simulink model "F16ASYM_Controlled_AoA"  (R2012b)
settings: Solver=ode3  SolverMode=SingleTasking  StartTime=0.0  StopTime=inf  FixedStep=T_sim  RelTol=1e-3
InitFcn:
  | load('NN_c_weights_Last_stable.mat')
values from neighbouring files (symbols this model uses):
  K_b_AoA = params(3)    [Cost_function.m]
  K_b_q = params(4)    [Cost_function.m]
  learning = 20    [Scheduling_desing.m]
  Model_used_flag = 1    [Scheduling_desing.m]
  reg_param = 0.5    [Scheduling_desing.m]
  T_sim = 0.02    [Scheduling_desing.m]
  tau_AoA = params(1)    [Cost_function.m]
  tau_q = params(2)    [Cost_function.m]
  Theta_1_roll_last = [0.00183613313267 0.00115998993235 0.0006676025148 0.00194921904952 0.00134963559861 0.00034352059664 0.000447169388141 0.00146749660935 0.00110199952389 7.77922383894e-05 0.00109492833348 0.00192687590535 ... (360 elements, 30x12)]    [NN_i_weights_LAST_STABLE.mat]
  Theta_2_roll_last = [0.000469743069697 0.000355923851088 0.00180035760697 0.00191855117771 0.00118851504447 0.0013331642065 0.0013164316578 0.000643981263341 0.00176817665434 0.000113802099363 0.000426534542462 0.00113815782354 ... (620 elements, 20x31)]    [NN_i_weights_LAST_STABLE.mat]
  Theta_3_roll_last = [9.62071520568e-05 -0.000389870886846 2.08260845013e-05 0.000140787743673 -0.000917525755397 -0.0014324207578 -0.00154701573815 -0.00131544476264 -0.00101205584381 5.06515794689e-05 -0.00111443483676 -0.00143957416141 ... (21 elements, 1x21)]    [NN_i_weights_LAST_STABLE.mat]
  V_long_lastA_w_z = [0.352826086601 -0.253633004548 -0.642535042878 0.237749930435 -0.618390629538 0.858074761295 0.268211230628 -0.448715080196 -0.0406384631192 0.401147605577 0.60598427709 0.0500551915851 ... (300 elements, 30x10)]    [NN_i_weights_LAST_STABLE.mat]
  V_long_lastAoA = [0.0774300162379 0.0911421319631 0.0352371192557 0.0542170286952 0.0651171200844 0.0177112012707 0.0982957728448 0.000259994642558 0.0194724569123 0.0466321328252 0.0556687953852 0.0252668067142 ... (300 elements, 30x10)]    [NN_i_weights_LAST_STABLE.mat]
  V_roll_last = [0.0540918675943 0.0557493347212 0.0839792276608 0.0460576391794 0.0671229058124 0.100220403067 0.0722493281881 0.0648875457457 0.00447599349201 0.0607299103823 0.0488037966361 0.0176785979393 ... (360 elements, 30x12)]    [NN_i_weights_LAST_STABLE.mat]
  V_yaw_last = [0.0965149149679 0.00833616709545 0.0365734360076 0.0523944217566 0.00790252078455 0.0700053845887 0.0345164868709 0.0111568465295 0.094060639546 0.0205483560006 0.000798047494256 0.0862769385758 ... (360 elements, 30x12)]    [NN_i_weights_LAST_STABLE.mat]
  velocity = M_eval_sche(I,J)*a    [Scheduling_desing.m]
  W_long_lastA_w_z = [-0.0522913429974 0.00385484301394 -0.00465489482472 -0.0139416219936 0.00295196421483 -0.013027768541 0.00585545058915 0.00278802233571 -0.00906272782329 -0.000396112031465 0.00405849743321 0.00509668457818 ... (31 elements, 1x31)]    [NN_i_weights_LAST_STABLE.mat]
  W_long_lastAoA = [-0.0192589013922 0.00873109909713 0.00432649597332 0.0420946902441 0.0293366820194 0.0351497798191 0.0234952374236 0.0360841187718 0.0112233388211 0.030147202199 0.0369533138617 0.00218839076415 ... (31 elements, 1x31)]    [NN_i_weights_LAST_STABLE.mat]
  W_roll_last = [-0.0006515532842 0.000535485585715 0.000550946920743 0.000806030945453 0.00045976209382 0.00065557954304 0.000945902185602 0.00070191398535 0.000635215543728 4.66501377412e-05 0.000597079583757 0.000485790566765 ... (31 elements, 1x31)]    [NN_i_weights_LAST_STABLE.mat]
  W_yaw_last = [-4.34263633305e-05 8.83823048922e-05 1.65575463724e-05 3.60293102233e-05 5.19752447623e-05 7.06399280852e-06 7.02425975821e-05 3.62680255076e-05 1.29996379937e-05 8.05072914397e-05 2.39941870661e-05 2.52427840574e-06 ... (31 elements, 1x31)]    [NN_i_weights_LAST_STABLE.mat]
undefined symbols (not defined in the file or in its folder): a1, alpha_map_eval, B, beta_map_eval, C_L_0, DiscIntNeverNeededParam, fi_flag_Simulink, G_eval, H_sq, H_sq_autotrim, k_B, m_B, M_sq, M_sq_autotrim, sigbuilder_block, Stall_curve, trim_control, trim_state, trim_throttle, V_Comp_A_w_z_last, V_Comp_last, V_roll_lastMOD, W_Comp_A_w_z_last, W_Comp_last, W_roll_lastMOD
libraries: Adaptive_FaultTolerantControl x43, dspsigops x29, F16_Actuator_Library x14, simulink x8, aerolibatmos2 x7, dsparch4 x6, simulink_extras x5, aerolibtransform2 x5, qcatlib x4, dspmtrx3 x3, dspvision x2, dspsnks4 x2
(part 11 of 11)

== matlab function F16ASYM_Controlled_AoA/Primary Controller/P controller + adaptive Isolated NN/On-line (adaptive) multi-layer NNs/Yaw Chanel/Yaw HL NN/Yaw NN ==
  data: X_bar input size=[12,1]; v_ad_comp output; e input; Ks input; B input; Long_learnign_rate input size=1; Long_reg_param input size=1; W input size=[1,31]; V input size=[30,12]; v_ad output; Z_norm_unit output; T_sim parameter; W_update output; V_update output
function [v_ad_comp,v_ad,Z_norm_unit,W_update,V_update]  = Yaw_NN(X_bar,e, Ks,B,Long_learnign_rate,Long_reg_param,W,V,T_sim)

%% Compute prelimiary parametes Ks(1)=K_b_alpha  and Ks(2) = K_b_q
P = [   1/Ks(1) , 1/(Ks(1)^2+Ks(1)*Ks(2));
     1/(Ks(1)^2+Ks(1)*Ks(2)) ,(Ks(1)^2+Ks(1)*Ks(2)+1)/(Ks(2)^2*Ks(1)+Ks(2)*Ks(1)^2) ];
zeta= e'*P*B;
s=zeros(30,1);
z=s;
%% Feedforward
z = V*X_bar;
s=sigmoid(V*X_bar);

sigma = [1 ; s ];
% v_ad = W*sigma;

sigma_grad = (sigma.*(ones(size(sigma))-sigma));

%% Compute the gradients or adaptation laws
Gamma_w= Long_learnign_rate; % W learnign rate
Gamma_v= Long_learnign_rate; %V learning rate
lambda = Long_reg_param;

V_dot=zeros(size(V));
W_dot=zeros(size(W'));

W_dot= -Gamma_w*(  (sigma - sigma_grad.*[1;z] ).*zeta  );
W_dot(2:end,1)= W_dot(2:end,1) - Gamma_w*lambda*norm(zeta)*(W(:,2:end))';

M = W'*zeta.*sigma_grad ;
V_dot= -Gamma_v*( M(2:end)*X_bar'  );
V_dot(:,2:end)= V_dot(:,2:end) - Gamma_v*lambda*norm(zeta).*V(:,2:end);


% % % Other way: Based on notes of Andrew NG
% % W_dot=zeros(size(W));
% % delta2=W'*zeta.*sigma_grad;
% % 
% % V_dot = - Gamma_v*( delta2(2:end)*X_bar');
% % V_dot(:,2:end)= V_dot(:,2:end) - Gamma_v*lambda*norm(zeta).*V(:,2:end);
% % 
% % W_dot = - Gamma_w*( zeta*sigma');
% % W_dot(:,2:end)= W_dot(:,2:end) - Gamma_w*lambda*norm(zeta)*(W(:,2:end));
% % 
% % W_dot = W_dot';


%% Adaptation
W_update = W + T_sim*W_dot';
V_update = V + T_sim*V_dot;

%% re-compute v_ad

z = V*X_bar;
s=sigmoid(V*X_bar);

sigma = [1 ; s(:,1) ];
v_ad = W*sigma;

%% Compute v_ad_comp
Z = [ V,zeros(size(V,1),size(W,2));
    zeros(size(W,1),size(V,2)),W];
    
Z_norm = norm(Z,'fro');
Z_max = 2*min(size(W,1),size(W,2) )*min( size(V,1),size(V,2) );
Z_norm_unit = Z_norm;

K_r0= 0.02;
K_r1= 0;
v_r0 = -K_r0*zeta;
v_r1 = -K_r1*(Z_norm+Z_max)*zeta;

v_ad_comp = v_ad + v_r1 +v_r0;


end

== matlab function F16ASYM_Controlled_AoA/NDI/NDI: RECONFIG/Pre-Inverter ==
  data: p_dot_comm input; L_comm output; q_dot_comm input; r_dot_comm input; M_comm output; N_comm output; omega_b input
function [L_comm,M_comm,N_comm] = Pre_inverter(p_dot_comm,q_dot_comm,r_dot_comm,omega_b)
Jy  = 75673.6;
Jxz = 1331.4; 
Jz  = 85552.1;  
Jx  = 12874.8;
h_E = 216.9;

Gamma = Jx * Jz - (Jxz  * Jxz);
C1 = ((Jy - Jz)  * Jz  - (Jxz * Jxz))/ Gamma;
C2 = ((Jx - Jy + Jz ) * Jxz ) / Gamma;
C3 = Jz / Gamma;
C4 = Jxz / Gamma;
C5 = (Jz - Jx) / Jy;
C6 = Jxz / Jy ;
C7 = 1 / Jy;
C8 = (Jx * (Jx - Jy ) + Jxz * Jxz) / Gamma;
C9 = Jx / Gamma;



L_comm = -( C4*r_dot_comm+(C2*C9-C4*C8)*omega_b(1)*omega_b(2)+(C2*C4+C1*C9)*omega_b(2)*omega_b(3)-C9*p_dot_comm )/(C3*C9-C4^2);

M_comm = (q_dot_comm-C5*omega_b(1)*omega_b(3)+C6*omega_b(1)^2-C6*omega_b(3)^2 +C7*h_E*omega_b(3))/C7;

N_comm = ( C3*r_dot_comm-C4*p_dot_comm+(C4*C1+C3*C2)*omega_b(2)*omega_b(3)+(C4*C2-C3*C8)*omega_b(1)*omega_b(2)+(C4^2-C3*C9)*h_E*omega_b(2) )/(C3*C9-C4^2);

== matlab function F16ASYM_Controlled_AoA/Primary Controller/P controller + adaptive Isolated NN/On-line (adaptive) multi-layer NNs SIMPL/Long Chanel/Long HL NN A_w_z/Long NN ==
  data: X_bar input size=[10,1]; v_ad_comp output; e input; F input; Ks input; B input; Long_learnign_rate input size=1; Long_reg_param input size=1; W input size=[1,31]; V input size=[30,10]; v_ad output; Z_norm_unit output; T_sim parameter; W_update output; V_update output
function [v_ad_comp,v_ad,Z_norm_unit,W_update,V_update]  = Long_AoA_NN(X_bar,e, F, Ks,B,Long_learnign_rate,Long_reg_param,W,V,T_sim)

%% Compute prelimiary parametes Ks(1)=K_b_alpha  and Ks(2) = K_b_q
P = [   1/Ks(1) , F/(Ks(1)^2+Ks(1)*Ks(2));
     1/(Ks(1)^2+Ks(1)*Ks(2)) ,(Ks(1)^2+Ks(1)*Ks(2)+F^2)/(Ks(2)^2*Ks(1)+Ks(2)*Ks(1)^2) ];
zeta= e'*P*B;
s=zeros(30,1);
z=s;
%% Feedforward
z = V*X_bar;
s=sigmoid(V*X_bar);

sigma = [1 ; s ];
% v_ad = W*sigma;

sigma_grad = (sigma.*(ones(size(sigma))-sigma));

%% Compute the gradients or adaptation laws
Gamma_w= Long_learnign_rate; % W learnign rate
Gamma_v= Long_learnign_rate; %V learning rate
lambda = Long_reg_param;

V_dot=zeros(size(V));
W_dot=zeros(size(W'));

W_dot= -Gamma_w*(  (sigma - sigma_grad.*[1;z] ).*zeta  );
W_dot(2:end,1)= W_dot(2:end,1) - Gamma_w*lambda*norm(zeta)*(W(:,2:end))';

M = W'*zeta.*sigma_grad ;
V_dot= -Gamma_v*( M(2:end)*X_bar'  );
V_dot(:,2:end)= V_dot(:,2:end) - Gamma_v*lambda*norm(zeta).*V(:,2:end);


% % % Other way: Based on notes of Andrew NG
% % W_dot=zeros(size(W));
% % delta2=W'*zeta.*sigma_grad;
% % 
% % V_dot = - Gamma_v*( delta2(2:end)*X_bar');
% % V_dot(:,2:end)= V_dot(:,2:end) - Gamma_v*lambda*norm(zeta).*V(:,2:end);
% % 
% % W_dot = - Gamma_w*( zeta*sigma');
% % W_dot(:,2:end)= W_dot(:,2:end) - Gamma_w*lambda*norm(zeta)*(W(:,2:end));
% % 
% % W_dot = W_dot';


%% Adaptation
W_update = W + T_sim*W_dot';
V_update = V + T_sim*V_dot;

%% re-compute v_ad

z = V*X_bar;
s=sigmoid(V*X_bar);

sigma = [1 ; s(:,1) ];
v_ad = W*sigma;

%% Compute v_ad_comp
Z = [ V,zeros(size(V,1),size(W,2));
    zeros(size(W,1),size(V,2)),W];
    
Z_norm = norm(Z,'fro');
Z_max = 2*min(size(W,1),size(W,2) )*min( size(V,1),size(V,2) );
Z_norm_unit = Z_norm/Z_max;

K_r0= 0.1;
K_r1= 0.001;
v_r0 = -K_r0*zeta;
v_r1 = -K_r1*(Z_norm+Z_max)*zeta;

v_ad_comp = v_ad + v_r1 +v_r0;


end

== matlab function F16ASYM_Controlled_AoA/Primary Controller/P controller + adaptive Isolated NN/On-line (adaptive) multi-layer NNs SIMPL/Long Chanel/Long HL NN AoA/Long NN ==
  data: X_bar input size=[10,1]; v_ad_comp output; e input; Ks input; B input; Long_learnign_rate input size=1; Long_reg_param input size=1; W input size=[1,31]; V input size=[30,10]; v_ad output; Z_norm_unit output; T_sim parameter; W_update output; V_update output
function [v_ad_comp,v_ad,Z_norm_unit,W_update,V_update]  = Long_AoA_NN(X_bar,e, Ks,B,Long_learnign_rate,Long_reg_param,W,V,T_sim)

%% Compute prelimiary parametes Ks(1)=K_b_alpha  and Ks(2) = K_b_q
P = [   1/Ks(1) , 1/(Ks(1)^2+Ks(1)*Ks(2));
     1/(Ks(1)^2+Ks(1)*Ks(2)) ,(Ks(1)^2+Ks(1)*Ks(2)+1)/(Ks(2)^2*Ks(1)+Ks(2)*Ks(1)^2) ];
zeta= e'*P*B;
s=zeros(30,1);
z=s;
%% Feedforward
z = V*X_bar;
s=sigmoid(V*X_bar);

sigma = [1 ; s ];
% v_ad = W*sigma;

sigma_grad = (sigma.*(ones(size(sigma))-sigma));

%% Compute the gradients or adaptation laws
Gamma_w= Long_learnign_rate; % W learnign rate
Gamma_v= Long_learnign_rate; %V learning rate
lambda = Long_reg_param;

V_dot=zeros(size(V));
W_dot=zeros(size(W'));

W_dot= -Gamma_w*(  (sigma - sigma_grad.*[1;z] ).*zeta  );
W_dot(2:end,1)= W_dot(2:end,1) - Gamma_w*lambda*norm(zeta)*(W(:,2:end))';

M = W'*zeta.*sigma_grad ;
V_dot= -Gamma_v*( M(2:end)*X_bar'  );
V_dot(:,2:end)= V_dot(:,2:end) - Gamma_v*lambda*norm(zeta).*V(:,2:end);


% % % Other way: Based on notes of Andrew NG
% % W_dot=zeros(size(W));
% % delta2=W'*zeta.*sigma_grad;
% % 
% % V_dot = - Gamma_v*( delta2(2:end)*X_bar');
% % V_dot(:,2:end)= V_dot(:,2:end) - Gamma_v*lambda*norm(zeta).*V(:,2:end);
% % 
% % W_dot = - Gamma_w*( zeta*sigma');
% % W_dot(:,2:end)= W_dot(:,2:end) - Gamma_w*lambda*norm(zeta)*(W(:,2:end));
% % 
% % W_dot = W_dot';


%% Adaptation
W_update = W + T_sim*W_dot';
V_update = V + T_sim*V_dot;

%% re-compute v_ad

z = V*X_bar;
s=sigmoid(V*X_bar);

sigma = [1 ; s(:,1) ];
v_ad = W*sigma;

%% Compute v_ad_comp
Z = [ V,zeros(size(V,1),size(W,2));
    zeros(size(W,1),size(V,2)),W];
    
Z_norm = norm(Z,'fro');
Z_max = 2*min(size(W,1),size(W,2) )*min( size(V,1),size(V,2) );
Z_norm_unit = Z_norm;

K_r0= 0.02;
K_r1= 0;
v_r0 = -K_r0*zeta;
v_r1 = -K_r1*(Z_norm+Z_max)*zeta;

v_ad_comp = v_ad + v_r1 +v_r0;


end

== matlab function F16ASYM_Controlled_AoA/Primary Controller/P controller + adaptive Isolated NN/On-line (adaptive) multi-layer NNs SIMPL/Roll NN/Roll 1HL NN/Roll NN ==
  data: X_bar input size=[8,1]; v_ad_comp output; e input; P input; B input; Roll_learnign_rate input size=1; Roll_reg_param input size=1; W input size=[1,31]; V input size=[30,8]; v_ad output; Z_norm_unit output; T_sim parameter; W_update output size=[1,31]; V_update output size=[30,8]
function [v_ad_comp,v_ad,Z_norm_unit,W_update,V_update]  = Roll_NN(X_bar,e,P,B,Roll_learnign_rate,Roll_reg_param,W,V,T_sim)

%% Compute prelimiary parametes
zeta= e'*P*B;
s=zeros(30,1);
z=s;
%% Feedforward
z = V*X_bar;
s=sigmoid(V*X_bar);

sigma = [1 ; s ];
% v_ad = W*sigma;

sigma_grad = (sigma.*(ones(size(sigma))-sigma));

%% Compute the gradients or adaptation laws
Gamma_w= Roll_learnign_rate; % W learnign rate
Gamma_v= Roll_learnign_rate; %V learning rate
lambda = Roll_reg_param;

V_dot=zeros(size(V));
W_dot=zeros(size(W'));

W_dot= -Gamma_w*(  (sigma - sigma_grad.*[1;z] ).*zeta  );
W_dot(2:end,1)= W_dot(2:end,1) - Gamma_w*lambda*norm(zeta)*(W(:,2:end))';

M = W'*zeta.*sigma_grad ;
V_dot= -Gamma_v*( M(2:end)*X_bar'  );
V_dot(:,2:end)= V_dot(:,2:end) - Gamma_v*lambda*norm(zeta).*V(:,2:end);


% Other way: Based on notes of Andrew NG
% % % % W_dot=zeros(size(W));
% % % % delta2=W'*zeta.*sigma_grad;
% % % % 
% % % % V_dot = - Gamma_v*( delta2(2:end)*X_bar');
% % % % V_dot(:,2:end)= V_dot(:,2:end) - Gamma_v*lambda*norm(zeta).*V(:,2:end);
% % % % 
% % % % W_dot = - Gamma_w*( zeta*sigma');
% % % % W_dot(:,2:end)= W_dot(:,2:end) - Gamma_w*lambda*norm(zeta)*(W(:,2:end));
% % % % 
% % % % W_dot = W_dot';


%% Adaptation
W_update = W + T_sim*W_dot';
V_update = V + T_sim*V_dot;

%% re-compute v_ad

z = V*X_bar;
s=sigmoid(V*X_bar);

sigma = [1 ; s(:,1) ];
v_ad = W*sigma;

%% Compute v_ad_comp
Z = [ V,zeros(size(V,1),size(W,2));
    zeros(size(W,1),size(V,2)),W];
    
Z_norm = norm(Z,'fro');
Z_max = 2*min(size(W,1),size(W,2) )*min( size(V,1),size(V,2) );
Z_norm_unit = Z_norm;

K_r0= 0;
K_r1= 0;
v_r0 = -K_r0*zeta;
v_r1 = -K_r1*(Z_norm+Z_max)*zeta;
v_ad_comp = v_ad + v_r1 +v_r0;

% % K_r1= 1;
% % v_r1 = - K_r1*(Z_norm+Z_max)*zeta;
% % 
% % v_ad_comp = v_ad + v_r1 ;



end

== matlab function F16ASYM_Controlled_AoA/Primary Controller/P controller + adaptive Isolated NN/On-line (adaptive) multi-layer NNs SIMPL/Roll NN/Roll 2HL NN/Roll Multilayer NN ==
  data: X_bar input size=[12,1]; v_ad_comp output; e input size=1; P input; B input; Roll_learnign_rate input size=1; Roll_reg_param input size=1; Theta_1 input size=[30,12]; Theta_2 input size=[20,31]; Theta_3 input size=[1,21]; v_ad output; Z_norm_unit output; T_sim parameter; Theta_1_update output; Theta_2_update output; Theta_3_update output
function [v_ad_comp,v_ad,Z_norm_unit,Theta_1_update,Theta_2_update,Theta_3_update]  = Roll_ML_NN(X_bar,e,P,B,Roll_learnign_rate, Roll_reg_param,Theta_1,Theta_2,Theta_3,T_sim)

%% Compute prelimiary parameters
zeta= e'*P*B;

%% Feedforward. Layers: Sigmoidal, linear, linear

a2=[1 ;  sigmoid( Theta_1*X_bar )]; % Sigmoidal
a3=[1 ;  (Theta_2*a2)]; % Linear
% z4=Theta_3*a3;
% a4 = z4; % Linear
% v_ad =a4;

% Backward
% % delta4=zeta; % In this particular case of adaptive NN, this error is a weighted tracking error
delta3=Theta_3'*zeta;
delta2=Theta_2'*delta3(2:end).*(a2.*(ones(size(a2))-a2)); 


%% Compute the gradients or adaptation laws
Gamma_Theta_3= Roll_learnign_rate; %  learnign rate
Gamma_Theta_2 = Roll_learnign_rate; % learning rate
Gamma_Theta_1= Roll_learnign_rate; % learning rate
lambda = Roll_reg_param;    % Regularization constant

% % Theta_1_dot=zeros(size(Theta_1));
% % Theta_2_dot=zeros(size(Theta_2));
% % Theta_3_dot=zeros(size(Theta_3));

Theta_3_dot = -Gamma_Theta_3*zeta*a3' ;
Theta_3_dot(:,2:end) =  Theta_3_dot(:,2:end) - Gamma_Theta_3*lambda*norm(zeta).*Theta_3(:,2:end);

Theta_2_dot= -Gamma_Theta_2*( delta3(2:end)*a2'   + lambda*norm(zeta).*Theta_2);
Theta_2_dot(:,2:end) =  Theta_2_dot(:,2:end) - Gamma_Theta_2*lambda*norm(zeta).*Theta_2(:,2:end);

Theta_1_dot= -Gamma_Theta_1*( delta2(2:end)*X_bar'   + lambda*norm(zeta).*Theta_1);
Theta_1_dot(:,2:end) =  Theta_1_dot(:,2:end) - Gamma_Theta_1*lambda*norm(zeta).*Theta_1(:,2:end);


%% Adaptation
Theta_1_update = Theta_1 + T_sim*Theta_1_dot;
Theta_2_update = Theta_2 + T_sim*Theta_2_dot;
Theta_3_update = Theta_3 + T_sim*Theta_3_dot;

%% re-compute v_ad

a2=[1 ;  sigmoid( Theta_1_update*X_bar )]; % Sigmoidal
a3=[1 ;  (Theta_2_update*a2)]; % Linear
v_ad=Theta_3_update*a3;


%% Compute v_ad_comp
% Z = blkdiag( Theta_1_update , Theta_2_update , Theta_3_update );

Z =  [ Theta_1_update, zeros(size(Theta_1_update,1),size(Theta_2_update,2)) , zeros(size(Theta_1_update,1),size(Theta_3_update,2));
            zeros(size(Theta_2_update,1),size(Theta_1_update,2)) , Theta_2_update , zeros(size(Theta_2_update,1),size(Theta_3_update,2)) ;
            zeros(size(Theta_3_update,1),size(Theta_1_update,2)),zeros(size(Theta_3_update,1),size(Theta_2_update,2)),  Theta_3_update ];

Z_norm = norm(Z,'fro');
Z_max = min(size(Theta_1))*min(size(Theta_2))*min(size(Theta_3));
Z_norm_unit = Z_norm;

K_r0= 0.02;
K_r1= 0;
v_r0 = -K_r0*zeta;
v_r1 = -K_r1*(Z_norm+Z_max)*zeta;

v_ad_comp = v_ad + v_r1 +v_r0;


end

== matlab function F16ASYM_Controlled_AoA/Primary Controller/P controller + adaptive Isolated NN/On-line (adaptive) multi-layer NNs SIMPL/Yaw Chanel/Yaw HL NN/Yaw NN ==
  data: X_bar input size=[12,1]; v_ad_comp output; e input; Ks input; B input; Long_learnign_rate input size=1; Long_reg_param input size=1; W input size=[1,31]; V input size=[30,12]; v_ad output; Z_norm_unit output; T_sim parameter; W_update output; V_update output
function [v_ad_comp,v_ad,Z_norm_unit,W_update,V_update]  = Yaw_NN(X_bar,e, Ks,B,Long_learnign_rate,Long_reg_param,W,V,T_sim)

%% Compute prelimiary parametes Ks(1)=K_b_alpha  and Ks(2) = K_b_q
P = [   1/Ks(1) , 1/(Ks(1)^2+Ks(1)*Ks(2));
     1/(Ks(1)^2+Ks(1)*Ks(2)) ,(Ks(1)^2+Ks(1)*Ks(2)+1)/(Ks(2)^2*Ks(1)+Ks(2)*Ks(1)^2) ];
zeta= e'*P*B;
s=zeros(30,1);
z=s;
%% Feedforward
z = V*X_bar;
s=sigmoid(V*X_bar);

sigma = [1 ; s ];
% v_ad = W*sigma;

sigma_grad = (sigma.*(ones(size(sigma))-sigma));

%% Compute the gradients or adaptation laws
Gamma_w= Long_learnign_rate; % W learnign rate
Gamma_v= Long_learnign_rate; %V learning rate
lambda = Long_reg_param;

V_dot=zeros(size(V));
W_dot=zeros(size(W'));

W_dot= -Gamma_w*(  (sigma - sigma_grad.*[1;z] ).*zeta  );
W_dot(2:end,1)= W_dot(2:end,1) - Gamma_w*lambda*norm(zeta)*(W(:,2:end))';

M = W'*zeta.*sigma_grad ;
V_dot= -Gamma_v*( M(2:end)*X_bar'  );
V_dot(:,2:end)= V_dot(:,2:end) - Gamma_v*lambda*norm(zeta).*V(:,2:end);


% % % Other way: Based on notes of Andrew NG
% % W_dot=zeros(size(W));
% % delta2=W'*zeta.*sigma_grad;
% % 
% % V_dot = - Gamma_v*( delta2(2:end)*X_bar');
% % V_dot(:,2:end)= V_dot(:,2:end) - Gamma_v*lambda*norm(zeta).*V(:,2:end);
% % 
% % W_dot = - Gamma_w*( zeta*sigma');
% % W_dot(:,2:end)= W_dot(:,2:end) - Gamma_w*lambda*norm(zeta)*(W(:,2:end));
% % 
% % W_dot = W_dot';


%% Adaptation
W_update = W + T_sim*W_dot';
V_update = V + T_sim*V_dot;

%% re-compute v_ad

z = V*X_bar;
s=sigmoid(V*X_bar);

sigma = [1 ; s(:,1) ];
v_ad = W*sigma;

%% Compute v_ad_comp
Z = [ V,zeros(size(V,1),size(W,2));
    zeros(size(W,1),size(V,2)),W];
    
Z_norm = norm(Z,'fro');
Z_max = 2*min(size(W,1),size(W,2) )*min( size(V,1),size(V,2) );
Z_norm_unit = Z_norm;

K_r0= 0.02;
K_r1= 0;
v_r0 = -K_r0*zeta;
v_r1 = -K_r1*(Z_norm+Z_max)*zeta;

v_ad_comp = v_ad + v_r1 +v_r0;


end

== matlab function F16ASYM_Controlled_AoA/Control allocator/Control allocator: RECONFIG/MATLAB Function ==
  data: Deflections input; Saturations output; Sup_lim input; Inf_lim input
function Saturations = Saturations(Deflections,Sup_lim,Inf_lim)
Saturations=zeros(7,1);

for i=1:7
    
    if Deflections(i)>=Sup_lim(i)
        Saturations(i)=1;
    elseif Deflections(i)<=Inf_lim(i)
        Saturations(i)=-1;
    else
        Saturations(i)=0;
    end
end

== matlab function F16ASYM_Controlled_AoA/Primary Controller/P controller + adaptive Crossed NN/Complete crossed On-line (adaptive) multi-layer NN/Complete crossed On-line (adaptive) multi-layer NN: A_w_z/Cross NN A_w_z ==
  data: X_bar input size=[25,1]; v_ad_comp output; e input; Factor_F input; K_roll input; Ks_long input; Ks_yaw input; B input; Learnign_rate input size=1; Reg_param input size=1; W input size=[3,51]; V input size=[50,25]; v_ad output; Z_norm_unit output; T_sim parameter; W_update output; V_update output
function [v_ad_comp,v_ad,Z_norm_unit,W_update,V_update]  = Cross_NN(X_bar,e,Factor_F, K_roll,Ks_long,Ks_yaw,B,Learnign_rate,Reg_param,W,V,T_sim)

%% Compute prelimiary parametes
% Compute P with regular Lyapunov equation solution
P_roll=1/K_roll;
P_long =  [   1/Ks_long(1) , Factor_F/(Ks_long(1)^2+Ks_long(1)*Ks_long(2));
     1/(Ks_long(1)^2+Ks_long(1)*Ks_long(2)) ,(Ks_long(1)^2+Ks_long(1)*Ks_long(2)+Factor_F^2)/(Ks_long(2)^2*Ks_long(1)+Ks_long(2)*Ks_long(1)^2) ];
P_yaw = [   1/Ks_yaw(1) , 1/(Ks_yaw(1)^2+Ks_yaw(1)*Ks_yaw(2));
     1/(Ks_yaw(1)^2+Ks_yaw(1)*Ks_yaw(2)) ,(Ks_yaw(1)^2+Ks_yaw(1)*Ks_yaw(2)+1)/(Ks_yaw(2)^2*Ks_yaw(1)+Ks_yaw(2)*Ks_yaw(1)^2) ];
 
P = blkdiag(P_roll,P_long,P_yaw);

% % % % Compute P with on-line Lyapunov equation solution
% % % CROSS = 0;
% % % A = [ -K_roll,0,CROSS,0,0;0,-Ks_long(1),1,0,0;
% % %     0,0,-Ks_long(2),0,0;0,0,0,-Ks_yaw(1),Factor_F;0,0,0,0,-Ks_yaw(2)];
% % % 
% % % coder.extrinsic('lyap')
% % % P = A;
% % % P = lyap(A,2*diag(ones(5,1)));



zeta= e'*P*B;

%% Feedforward
z = V*X_bar;
s=sigmoid(V*X_bar);

sigma = [1 ; s ];
% v_ad = W*sigma;

sigma_grad = (sigma.*(ones(size(sigma))-sigma));

%% Compute the gradients or adaptation laws
Gamma_w= Learnign_rate; % W learnign rate
Gamma_v= Learnign_rate; %V learning rate
lambda = Reg_param;

V_dot=zeros(size(V));
W_dot=zeros(size(W));

W_dot= -Gamma_w*(  (sigma - sigma_grad.*[1;z] )*zeta  )';
W_dot(:,2:end)= W_dot(:,2:end) - Gamma_w*lambda*norm(zeta)*(W(:,2:end));

M = W'*zeta'.*sigma_grad ;
V_dot= -Gamma_v*( M(2:end)*X_bar'  );
V_dot(:,2:end)= V_dot(:,2:end) - Gamma_v*lambda*norm(zeta).*V(:,2:end);

% % % % 
% % % % % Other way: Based on notes of Andrew NG
% % % % 
% % % % delta2=W'*zeta'.*sigma_grad;
% % % % 
% % % % V_dot = - Gamma_v*( delta2(2:end)*X_bar');
% % % % V_dot(:,2:end)= V_dot(:,2:end) - Gamma_v*lambda*norm(zeta).*V(:,2:end);
% % % % 
% % % % W_dot = - Gamma_w*( sigma*zeta)';
% % % % W_dot(:,2:end)= W_dot(:,2:end) - Gamma_w*lambda*norm(zeta)*(W(:,2:end));



%% Adaptation
W_update = W + T_sim*W_dot;
V_update = V + T_sim*V_dot;

%% Re-compute v_ad

s=sigmoid(V_update*X_bar);

sigma = [1 ; s(:,1) ];
v_ad = W_update*sigma;

%% Compute v_ad_comp
Z = [ V,zeros(size(V,1),size(W,2));
    zeros(size(W,1),size(V,2)),W];
    
Z_norm = norm(Z,'fro');
Z_max = 2*min(size(W,1),size(W,2) )*min( size(V,1),size(V,2) );
Z_norm_unit = Z_norm;

K_r0= 0.02;
K_r1= 0;
v_r0 = -K_r0*zeta';
v_r1 = -K_r1*(Z_norm+Z_max)*zeta';

v_ad_comp = v_ad + v_r1 +v_r0;


end

== matlab function F16ASYM_Controlled_AoA/Primary Controller/P controller + adaptive Crossed NN/Sigmoid /MATLAB Function ==
  data: u input; y output; a input
function y = sigmoid_a(u,a)

y = 2.0 ./ (1.0 + exp(-a*u(1:3)))-1;

== matlab function F16ASYM_Controlled_AoA/Primary Controller/P controller + adaptive Crossed NN + AWU+Lim /Complete crossed On-line (adaptive) multi-layer NN/Complete crossed On-line (adaptive) multi-layer NN: A_w_z/Cross NN A_w_z ==
  data: X_bar input size=[25,1]; v_ad_comp output; e input; Factor_F input; K_roll input; Ks_long input; Ks_yaw input; B input; Learnign_rate input size=1; Reg_param input size=1; AWU input; W input size=[3,51]; V input size=[50,25]; v_ad output; Z_norm_unit output; T_sim parameter; W_update output; V_update output
function [v_ad_comp,v_ad,Z_norm_unit,W_update,V_update]  = Cross_NN(X_bar,e,Factor_F, K_roll,Ks_long,Ks_yaw,B,Learnign_rate,Reg_param,AWU,W,V,T_sim)

%% Compute prelimiary parametes
% Compute P with regular Lyapunov equation solution
P_roll=1/K_roll;
P_long =  [   1/Ks_long(1) , Factor_F/(Ks_long(1)^2+Ks_long(1)*Ks_long(2));
     1/(Ks_long(1)^2+Ks_long(1)*Ks_long(2)) ,(Ks_long(1)^2+Ks_long(1)*Ks_long(2)+Factor_F^2)/(Ks_long(2)^2*Ks_long(1)+Ks_long(2)*Ks_long(1)^2) ];
P_yaw = [   1/Ks_yaw(1) , 1/(Ks_yaw(1)^2+Ks_yaw(1)*Ks_yaw(2));
     1/(Ks_yaw(1)^2+Ks_yaw(1)*Ks_yaw(2)) ,(Ks_yaw(1)^2+Ks_yaw(1)*Ks_yaw(2)+1)/(Ks_yaw(2)^2*Ks_yaw(1)+Ks_yaw(2)*Ks_yaw(1)^2) ];
 
P = blkdiag(P_roll,P_long,P_yaw);

% % % % Compute P with on-line Lyapunov equation solution
% % % CROSS = 0;
% % % A = [ -K_roll,0,CROSS,0,0;0,-Ks_long(1),1,0,0;
% % %     0,0,-Ks_long(2),0,0;0,0,0,-Ks_yaw(1),Factor_F;0,0,0,0,-Ks_yaw(2)];
% % % 
% % % coder.extrinsic('lyap')
% % % P = A;
% % % P = lyap(A,2*diag(ones(5,1)));



K_awu = 1.2;
zeta= e'*P*B;


% Introduce Anti-windup
zeta = zeta - K_awu*AWU'.*T_sim; 

% Convergence limitation
if norm(zeta)>2/(T_sim*Learnign_rate*Reg_param)
    zeta = (zeta./norm(zeta)).*(1.8/(T_sim*Learnign_rate*Reg_param));
end

%% Feedforward
z = V*X_bar;
s=sigmoid(V*X_bar);

sigma = [1 ; s ];
% v_ad = W*sigma;

sigma_grad = (sigma.*(ones(size(sigma))-sigma));

%% Compute the gradients or adaptation laws
Gamma_w= Learnign_rate; % W learnign rate
Gamma_v= Learnign_rate; %V learning rate
lambda = Reg_param;

V_dot=zeros(size(V));
W_dot=zeros(size(W));

W_dot= -Gamma_w*(  (sigma - sigma_grad.*[1;z] )*zeta  )';
W_dot(:,2:end)= W_dot(:,2:end) - Gamma_w*lambda*norm(zeta)*(W(:,2:end));

M = W'*zeta'.*sigma_grad ;
V_dot= -Gamma_v*( M(2:end)*X_bar'  );
V_dot(:,2:end)= V_dot(:,2:end) - Gamma_v*lambda*norm(zeta).*V(:,2:end);

% % % Other way: Based on notes of Andrew NG
% % 
% % delta2=W'*zeta'.*sigma_grad;
% % 
% % V_dot = - Gamma_v*( delta2(2:end)*X_bar');
% % V_dot(:,2:end)= V_dot(:,2:end) - Gamma_v*lambda*norm(zeta).*V(:,2:end);
% % 
% % W_dot = - Gamma_w*( sigma*zeta)';
% % W_dot(:,2:end)= W_dot(:,2:end) - Gamma_w*lambda*norm(zeta)*(W(:,2:end));



%% Adaptation
W_update = W + T_sim*W_dot;
V_update = V + T_sim*V_dot;
% 
%% Re-compute v_ad

s=sigmoid(V_update*X_bar);

sigma = [1 ; s(:,1) ];
v_ad = W_update*sigma;

%% Compute v_ad_comp
Z = [ V,zeros(size(V,1),size(W,2));
    zeros(size(W,1),size(V,2)),W];
    
Z_norm = norm(Z,'fro');
Z_max = 2*min(size(W,1),size(W,2) )*min( size(V,1),size(V,2) );
Z_norm_unit = Z_norm;

K_r0= 0;
K_r1= 0;
v_r0 = -K_r0*zeta';
v_r1 = -K_r1*(Z_norm+Z_max)*zeta';

v_ad_comp = v_ad + v_r1 +v_r0;

% % % Normalization of matrices
% % if Z_norm>Z_max
% %     V = (V.*Z_max)./Z_norm;
% %     W = (W.*Z_max)./Z_norm;
% % end
end
